simulink model "walkingRobot3DMPC"  (R2019b)
settings: Solver=ode15s  StartTime=0.0  StopTime=15  RelTol=1e-2  EnableMultiTasking=on
PreLoadFcn:
  | robotParametersCtrl
  | designMPCWalkingPatternGen
  | 
  | % Define trajectory points for visualization
  | interPts = [0 0 0; 1 0 0];
undefined symbols (not defined in the file): h, numOutputs, predictionHorizon, stepLength, stepTime, stepWidth, torso_y, Ts
libraries: walkingRobotUtils x4, cstblocks x2, mpclib x2, simulink x1
settings Model: Creator=scastro  LastModifiedBy=scastro
settings DataIOCC: ReturnWorkspaceOutputs=off  OutputTimes=0:0.01:10
settings OptimizationCC: LifeSpan=inf
settings DebuggingCC: AllowSymbolicDim=off  SFUnexpectedBacktrackingDiag=warning  SFNoUnconditionalDefaultTransitionDiag=warning  SFExecutionAtInitializationDiag=none  UnitsInconsistencyMsg=none  ArithmeticOperatorsInVariantConditions=warning
settings SFSimCC: SimUseLocalCustomCode=off  CustomCodeUndefinedFunction=UseInterfaceOnly
settings RTWCC: RTWUseLocalCustomCode=off
settings CodeAppCC: StateflowObjectComments=on
settings GRTTargetCC: TargetLangStandard=C89/C90 (ANSI)  GeneratePreprocessorConditionals=Disable all
settings ConfigComp: CovMetricSettings=dw  CovHtmlReporting=on  CovSaveCumulativeToWorkspaceVar=on  CovSaveSingleToWorkspaceVar=on  CovExternalEMLEnable=off  CovSFcnEnable=off
settings SimscapeCC: SimscapeNormalizeSystem=off  SimscapeLogOpenViewer=on  SimscapeLogLimitData=off  SimscapeLogDataHistory=10000
settings ConfigurationSet: Description=SimMechanics 2G
settings DiagnosticsConfigSet: SimMechanicsRigidlyBoundBlock=none
settings ExplorerConfigSet: InternalSimMechanicsExplorerSettings="<ExplorerConfiguration><canonicalview>default</canonicalview><AnimationSetting><BasePlaybackSpeed>1.0</BasePlaybackSpeed><PlaybackSpeedFactor>1.0</PlaybackSpeedFactor></AnimationSetting><TilePanel><TileInfo><Tiles Columns=\"1\" Count=\"1\" Rows=\"1\"><Column Weight=\"1\"/><Row Weight=\"1\"/><Tile Height=\"1\" Width=\"1\" X=\"0\" Y=\"0\"/></Tiles></TileInfo><SceneInfo><SceneViewer><BGColor><R>0.60000002384185791</R><G>0.60000002384185791</G><B>0.60000002384185791</B></BGColor><Camera><DoPerspective>off</DoPerspective><Position><X>7.18002534815406079</X><Y>-8.21011991112170847</Y><Z>8.33180938462712462</Z></Position><Center><X>1.10741005252516134</X><Y>-0.176829942633513204</Y><Z>0.646464709811595872</Z></Center><Up><X>-0.335329266167064488</X><Y>0.506481739462631531</Y><Z>0.79437430147428989</Z></Up><ViewLimDist>1</ViewLimDist><YLim>0.739205014828661411</YLim><XLim>1.12849377732657596</XLim></Camera></SceneViewer></SceneInfo></TilePanel><MechEditorPanel><Cameras/><GfxPanelCameraMap/><VideoCreator><PlaybackSpeedRatio>1.0</PlaybackSpeedRatio><FrameRate>30</FrameRate><VideoFormat>Motion JPEG AVI</VideoFormat><FrameSize>auto</FrameSize></VideoCreator></MechEditorPanel></ExplorerConfiguration>"

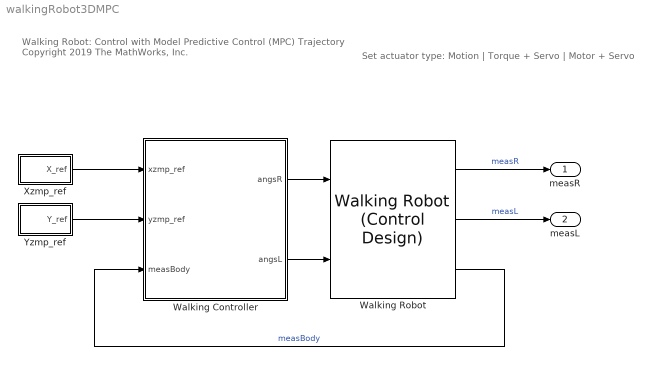
== system walkingRobot3DMPC ==
  note: Set actuator type:
      | Motion | Torque + Servo | Motor + Servo
  note: Walking Robot: Control with Model Predictive Control (MPC) Trajectory
      |
      | Copyright 2019 The MathWorks, Inc.
  Walking Controller : Subsystem
  Walking Robot : walkingRobotUtils/Walking Robot (Control Design)  SystemSampleTime=-1  Latency=0  AutoFrameSizeCalculation=off
  Xzmp_ref : Subsystem
  Yzmp_ref : Subsystem
  measR : Outport
  measL : Outport  Port=2
  wires:
  Walking Robot/1 -> measR/1  "measR"
  Walking Robot/2 -> measL/1  "measL"
  Walking Controller/1(angsR) -> Walking Robot/1
  Walking Controller/2(angsL) -> Walking Robot/2
  Walking Robot/3 -> Walking Controller/3(measBody)  "measBody"
  Yzmp_ref/1(Y_ref) -> Walking Controller/2(yzmp_ref)
  Xzmp_ref/1(X_ref) -> Walking Controller/1(xzmp_ref)

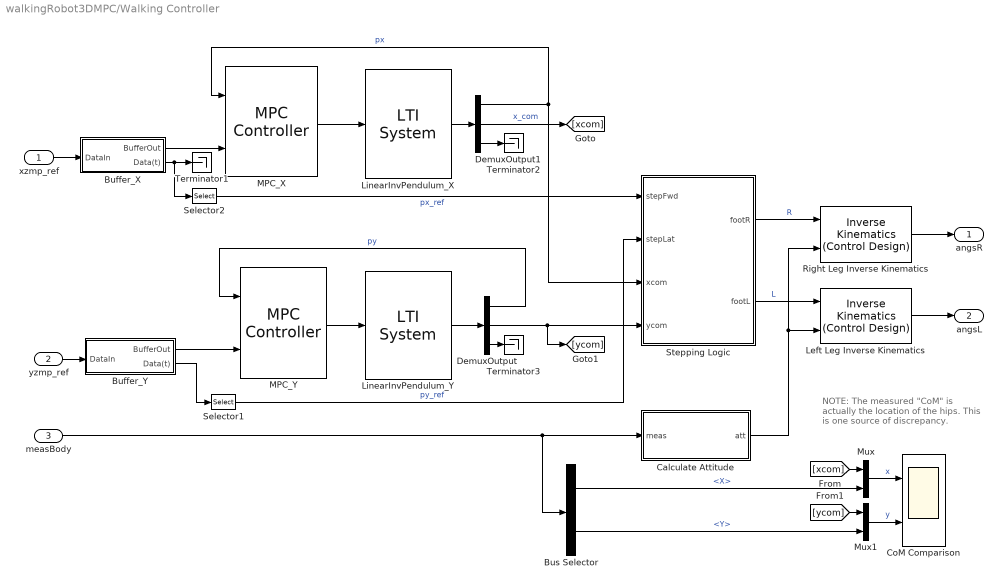
== system walkingRobot3DMPC/Walking Controller ==
  note: NOTE: The measured "CoM" is
      | actually the location of the hips.
      |
      | This is one source of discrepancy.
  xzmp_ref : Inport
  yzmp_ref : Inport  Port=2
  measBody : Inport  Port=3
  Buffer_X : Subsystem
  Buffer_Y : Subsystem
  Bus Selector : BusSelector  OutputSignals=X,Y
  Calculate Attitude : Subsystem
  CoM Comparison : Scope  NumInputPorts=2
  DemuxOutput : Demux  Outputs=3
  DemuxOutput1 : Demux  Outputs=3
  Left Leg Inverse Kinematics : walkingRobotUtils/Inverse Kinematics (Control Design)  SystemSampleTime=-1  Latency=0  AutoFrameSizeCalculation=off
  LinearInvPendulum_X : cstblocks/LTI System  sys=lip_x_d  IC=[0;0;0]  mask(LTI Block){}
      mask Display:
      | % This is a new mask on top of the base mask.
      | % Use "View base mask" link below to see the base mask.
      | image('lipm.jpg')
  LinearInvPendulum_Y : cstblocks/LTI System  sys=lip_y_d  IC=[0;0;0]  mask(LTI Block){}
      mask Display:
      | % This is a new mask on top of the base mask.
      | % Use "View base mask" link below to see the base mask.
      | image('lipm.jpg');
  MPC_X : mpclib/MPC Controller  SCDEnableBlockLinearizationSpecification=on  mpcobj=mpc1  is_multiple=0  enable_value=0  return_u0=off  updateMPCinCallerWorkspace=on  md_inport=off  mv_inport=off  uref_inport=off  return_cost=off  return_mvseq=off  return_qpstatus=off  return_xseq=off  return_state=off  return_ovseq=off  state_inport=off  umin_inport=off  umax_inport=off  ymin_inport=off  ymax_inport=off  cc_inport=off  ywt_inport=off  uwt_inport=off  duwt_inport=off  rhoeps_inport=off  pm_inport=off  MaximumP=10  HorizonChoice=FixedHorizon  n_ts=0.01  n_p=50  n_mv=1  n_md=0  n_ud=0  n_mo=1  n_uo=2  BlockDataType=double  SampleTimeInherited=off  switch_inport=off
  MPC_Y : mpclib/MPC Controller  SCDEnableBlockLinearizationSpecification=on  mpcobj=mpc1  is_multiple=0  enable_value=0  return_u0=off  updateMPCinCallerWorkspace=on  md_inport=off  mv_inport=off  uref_inport=off  return_cost=off  return_mvseq=off  return_qpstatus=off  return_xseq=off  return_state=off  return_ovseq=off  state_inport=off  umin_inport=off  umax_inport=off  ymin_inport=off  ymax_inport=off  cc_inport=off  ywt_inport=off  uwt_inport=off  duwt_inport=off  rhoeps_inport=off  pm_inport=off  MaximumP=10  HorizonChoice=FixedHorizon  n_ts=0.01  n_p=50  n_mv=1  n_md=0  n_ud=0  n_mo=1  n_uo=2  BlockDataType=double  SampleTimeInherited=off  switch_inport=off
  Mux : Mux  Inputs=2
  Mux1 : Mux  Inputs=2
  Right Leg Inverse Kinematics : walkingRobotUtils/Inverse Kinematics (Control Design)  SystemSampleTime=-1  Latency=0  AutoFrameSizeCalculation=off
  Selector1 : Selector  InputPortWidth=3  IndexOptions=Index vector (dialog)  Indices=[1]  OutputSizes=1
  Selector2 : Selector  InputPortWidth=3  IndexOptions=Index vector (dialog)  Indices=[1]  OutputSizes=1
  Stepping Logic : Stateflow chart  TreatAsAtomicUnit=on
  Terminator1 : Terminator
  Terminator2 : Terminator
  Terminator3 : Terminator
  angsR : Outport
  angsL : Outport  Port=2
  wires:
  Stepping Logic/1(footR) -> Right Leg Inverse Kinematics/1  "R"
  Stepping Logic/2(footL) -> Left Leg Inverse Kinematics/1  "L"
  Buffer_X/1(BufferOut) -> MPC_X/2
  LinearInvPendulum_X/1 -> DemuxOutput1/1
  xzmp_ref/1 -> Buffer_X/1(DataIn)
  MPC_X/1 -> LinearInvPendulum_X/1
  DemuxOutput1/1 -> Stepping Logic/3(xcom), MPC_X/1  "px"
  Buffer_X/2(Data(t)) -> Selector2/1, Terminator1/1
  LinearInvPendulum_Y/1 -> DemuxOutput/1
  yzmp_ref/1 -> Buffer_Y/1(DataIn)
  Buffer_Y/1(BufferOut) -> MPC_Y/2
  MPC_Y/1 -> LinearInvPendulum_Y/1
  Buffer_Y/2(Data(t)) -> Selector1/1
  DemuxOutput/1 -> MPC_Y/1  "py"
  measBody/1 -> Bus Selector/1, Calculate Attitude/1(meas)
  Calculate Attitude/1(att) -> Right Leg Inverse Kinematics/2, Left Leg Inverse Kinematics/2
  Right Leg Inverse Kinematics/1 -> angsR/1
  Left Leg Inverse Kinematics/1 -> angsL/1
  DemuxOutput1/3 -> Terminator2/1
  DemuxOutput/3 -> Terminator3/1
  Bus Selector/1 -> Mux/2  "<X>"
  Bus Selector/2 -> Mux1/2  "<Y>"
  DemuxOutput1/2 -> [xcom]  "x_com"
  DemuxOutput/2 -> [ycom], Stepping Logic/4(ycom)
  Selector1/1 -> Stepping Logic/2(stepLat)  "py_ref"
  Mux/1 -> CoM Comparison/1  "x"
  Mux1/1 -> CoM Comparison/2  "y"
  [xcom] -> Mux/1
  [ycom] -> Mux1/1
  Selector2/1 -> Stepping Logic/1(stepFwd)  "px_ref"

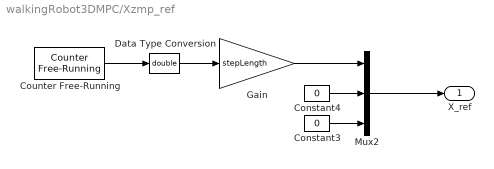
== system walkingRobot3DMPC/Xzmp_ref ==
  Constant3 : Constant  Value=0  SampleTime=Ts
  Constant4 : Constant  Value=0  SampleTime=Ts
  Counter Free-Running : simulink/Sources/Counter Free-Running  NumBits=64  tsamp=stepTime
  Data Type Conversion : DataTypeConversion  OutDataTypeStr=double
  Gain : Gain  Gain=stepLength
  Mux2 : Mux  Inputs=3
  X_ref : Outport
  wires:
  Gain/1 -> Mux2/1
  Constant3/1 -> Mux2/3
  Data Type Conversion/1 -> Gain/1
  Counter Free-Running/1 -> Data Type Conversion/1
  Mux2/1 -> X_ref/1
  Constant4/1 -> Mux2/2

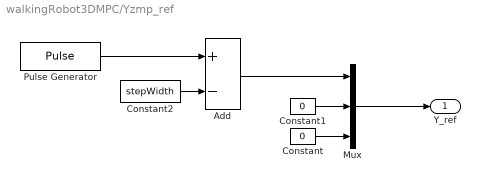
== system walkingRobot3DMPC/Yzmp_ref ==
  Add : Sum  Inputs=+-
  Constant : Constant  Value=0  SampleTime=Ts
  Constant1 : Constant  Value=0  SampleTime=Ts
  Constant2 : Constant  Value=stepWidth  SampleTime=Ts
  Mux : Mux  Inputs=3
  Pulse Generator : DiscretePulseGenerator  PulseType=Time based  Amplitude=2*stepWidth  Period=2*stepTime  PulseWidth=50
  Y_ref : Outport
  wires:
  Mux/1 -> Y_ref/1
  Constant1/1 -> Mux/2
  Constant2/1 -> Add/2
  Constant/1 -> Mux/3
  Add/1 -> Mux/1
  Pulse Generator/1 -> Add/1

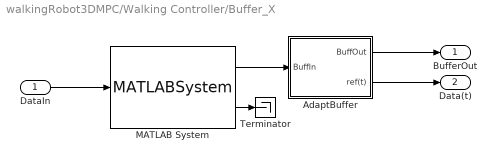
== system walkingRobot3DMPC/Walking Controller/Buffer_X ==
  DataIn : Inport
  AdaptBuffer : Subsystem
  MATLAB System : MATLABSystem  System=FIFOBuffer  Capacity=predictionHorizon  NumStates=numOutputs  SampleTime=Ts  FillBufferAtStartup=on  BufferStartupFillupData=zeros(numOutputs,predictionHorizon)  SimulateUsing=Code generation
      mask Type: FIFOBuffer
      mask Display:
      | disp('FIFOBuffer');
      | port_label('input',1,'dataIn');
      | port_label('output',1,'buffer');
      | port_label('output',2,'isFull');
  Terminator : Terminator
  BufferOut : Outport
  Data(t) : Outport  Port=2
  wires:
  AdaptBuffer/2(ref(t)) -> Data(t)/1
  DataIn/1 -> MATLAB System/1
  MATLAB System/2 -> Terminator/1
  AdaptBuffer/1(BuffOut) -> BufferOut/1
  MATLAB System/1 -> AdaptBuffer/1(BuffIn)

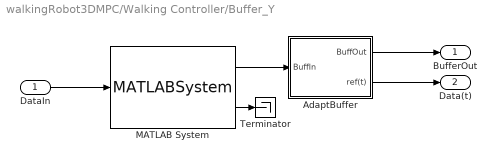
== system walkingRobot3DMPC/Walking Controller/Buffer_Y ==
  DataIn : Inport
  AdaptBuffer : Subsystem
  MATLAB System : MATLABSystem  System=FIFOBuffer  Capacity=predictionHorizon  NumStates=numOutputs  SampleTime=Ts  FillBufferAtStartup=on  BufferStartupFillupData=zeros(numOutputs,predictionHorizon)  SimulateUsing=Code generation
      mask Type: FIFOBuffer
      mask Display:
      | disp('FIFOBuffer');
      | port_label('input',1,'dataIn');
      | port_label('output',1,'buffer');
      | port_label('output',2,'isFull');
  Terminator : Terminator
  BufferOut : Outport
  Data(t) : Outport  Port=2
  wires:
  MATLAB System/1 -> AdaptBuffer/1(BuffIn)
  AdaptBuffer/1(BuffOut) -> BufferOut/1
  MATLAB System/2 -> Terminator/1
  DataIn/1 -> MATLAB System/1
  AdaptBuffer/2(ref(t)) -> Data(t)/1

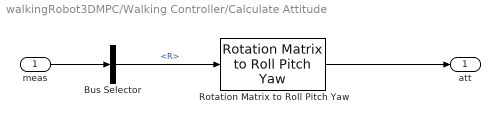
== system walkingRobot3DMPC/Walking Controller/Calculate Attitude ==
  meas : Inport
  Bus Selector : BusSelector  OutputSignals=R
  Rotation Matrix to Roll Pitch Yaw : walkingRobotUtils/Rotation Matrix to  Roll Pitch Yaw  SystemSampleTime=-1  Latency=0  AutoFrameSizeCalculation=off
      settings: SourceProductName=Simulink  SourceProductBaseCode=SL
  att : Outport
  wires:
  Bus Selector/1 -> Rotation Matrix to Roll Pitch Yaw/1  "<R>"
  meas/1 -> Bus Selector/1
  Rotation Matrix to Roll Pitch Yaw/1 -> att/1

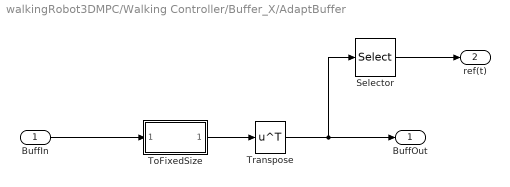
== system walkingRobot3DMPC/Walking Controller/Buffer_X/AdaptBuffer ==
  BuffIn : Inport
  Selector : Selector  NumberOfDimensions=2  InputPortWidth=3  IndexOptions=Index vector (dialog),Select all  Indices=[1],1  OutputSizes=1,1
  ToFixedSize : MATLAB Function  TreatAsAtomicUnit=on  mask{predictionHorizon=predictionHorizon, numStates=numOutputs}
      mask prompts: predictionHorizon "Prediction Horizon"; numStates "Number of States"
  Transpose : Math  Operator=transpose  SaturateOnIntegerOverflow=on
  BuffOut : Outport
  ref(t) : Outport  Port=2
  wires:
  Selector/1 -> ref(t)/1
  BuffIn/1 -> ToFixedSize/1(buffIn)
  Transpose/1 -> BuffOut/1, Selector/1
  ToFixedSize/1(buffOut) -> Transpose/1

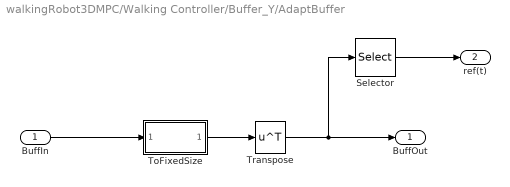
== system walkingRobot3DMPC/Walking Controller/Buffer_Y/AdaptBuffer ==
  BuffIn : Inport
  Selector : Selector  NumberOfDimensions=2  InputPortWidth=3  IndexOptions=Index vector (dialog),Select all  Indices=[1],1  OutputSizes=1,1
  ToFixedSize : MATLAB Function  TreatAsAtomicUnit=on  mask{predictionHorizon=predictionHorizon, numStates=numOutputs}
      mask prompts: predictionHorizon "Prediction Horizon"; numStates "Number of States"
  Transpose : Math  Operator=transpose  SaturateOnIntegerOverflow=on
  BuffOut : Outport
  ref(t) : Outport  Port=2
  wires:
  ToFixedSize/1(buffOut) -> Transpose/1
  Transpose/1 -> Selector/1, BuffOut/1
  BuffIn/1 -> ToFixedSize/1(buffIn)
  Selector/1 -> ref(t)/1

== matlab function walkingRobot3DMPC/Walking Controller/Buffer_X/AdaptBuffer/ToFixedSize ==
  data: buffIn input size=[numStates,predictionHorizon]; buffOut output size=[numStates,predictionHorizon]; predictionHorizon parameter size=1; numStates parameter size=1
function buffOut = fcn(buffIn,predictionHorizon, numStates)

buffOut = buffIn(1:numStates,1:predictionHorizon);

== matlab function walkingRobot3DMPC/Walking Controller/Buffer_Y/AdaptBuffer/ToFixedSize ==
  data: buffIn input size=[numStates,predictionHorizon]; buffOut output size=[numStates,predictionHorizon]; predictionHorizon parameter size=1; numStates parameter size=1
function buffOut = fcn(buffIn,predictionHorizon, numStates)

buffOut = buffIn(1:numStates,1:predictionHorizon);

== stateflow chart walkingRobot3DMPC/Walking Controller/Stepping Logic ==
  settings: updateMethod=DISCRETE
  state control [function]
    (default) -> (junction 43) : {
        | xR = xR + Kwalk*(xrefR-xR);
        | yR = yR + Kwalk*(yrefR-yR);
        | zR = zR + Kwalk*(zrefR-zR);
        | xL = xL + Kwalk*(xrefL-xL);
        | yL = yL + Kwalk*(yrefL-yL);
        | zL = zL + Kwalk*(zrefL-zL);
        | footR = [xR;yR;zR];
        | footL = [xL;yL;zL];
        | }
  state Wait
    en,du:
    control;
  state RightStep
    % Right foot is active
    % Left foot drags
    en, du:
    control;
    state RightFoot [parallel]
      en,du:
      zrefL = low;
      xrefR = stepFwd - xcom;
      yrefR = min(0,stepLat-(ycom-del));
      on after(0.05*stepTime,sec):
      zrefR = high;
      on after(0.95*stepTime,sec):
      zrefR = low;
      settings: executionOrder=2
    state LeftFoot [parallel]
      en:
      refsnap = [xrefL+xcom ...
      yrefL+ycom];
      en, du:
      xrefL = refsnap(1) - xcom;
      yrefL = max(0,refsnap(2) - ycom);
      settings: executionOrder=1
  state LeftStep
    % Left foot is active
    % Right foot drags
    en,du:
    control;
    state RightFoot [parallel]
      en:
      refsnap = [xrefR+xcom ...
      yrefR+ycom];
      en, du:
      xrefR = refsnap(1) - xcom;
      yrefR = min(0,refsnap(2) - ycom);
      settings: executionOrder=1
    state LeftFoot [parallel]
      en,du:
      zrefR = low;
      xrefL = stepFwd - xcom;
      yrefL =  max(0,stepLat-(ycom+del));
      on after(0.05*stepTime,sec):
      zrefL = high;
      on after(0.95*stepTime,sec):
      zrefL = low;
      settings: executionOrder=2
  (default) -> Wait : % Initialize values
      | {
      | Kwalk = 0.2; stepHeight = 0.01;
      | low = -h/100;
      | high = low + stepHeight;
      | xL = 0; yL = 0; zL = low;
      | xR = 0; yR = 0; zR = low;
      | xrefL = 0; yrefL = 0; zrefL = low;
      | xrefR = 0; yrefR = 0; zrefR = low;
      | del = torso_y/200;
      | }
  Wait -> (junction 83) : [after(stepTime/2,sec)]
  (junction 83) -> LeftStep
  RightStep -> LeftStep : %[after(stepTime,sec)]
      | [stepLat > 0]
  LeftStep -> RightStep : %[after(stepTime,sec)]
      | [stepLat < 0]
  data: footR output; footL output; stepFwd input; stepLat input; xR local; yR local; zR local; high local; xL local; yL local; zL local; low local; stepHeight local; h parameter; Kwalk local; yrefL local; zrefL local; xrefL local; yrefR local; zrefR local; xrefR local; stepTime parameter; xcom input; refsnap local; ycom input; torso_y parameter; del local
